simulink library "gbt_library"  (Simulink 7.4)
settings: Solver=ode45  StartTime=0.0  StopTime=10.0  RelTol=1e-3
undefined symbols (not defined in the file or in its folder): xlipgetpartsetting
libraries: xbsIndex_r4 x1348, casper_library_misc x29, casper_library_flow_control x4
(part 2 of 11)

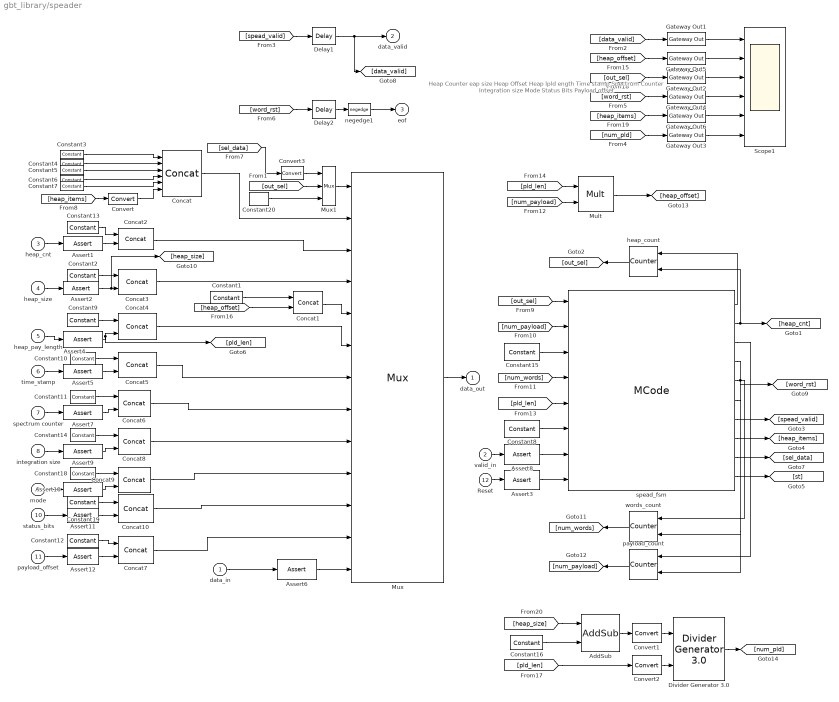
== system gbt_library/speader ==
  note: Heap Counter
      | eap size
      | Heap Offset
      | Heap lpld ength
      | Time stamp
      | Spectrum Counter
      | Integration size
      | Mode
      | Status Bits
      | Payload offset
  data_in : Inport
  valid_in : Inport  Port=2
  heap_cnt : Inport  Port=3
  heap_size : Inport  Port=4
  heap_pay_length : Inport  Port=5
  time_stamp : Inport  Port=6
  spectrum counter : Inport  Port=7
  integration size : Inport  Port=8
  mode : Inport  Port=9
  status_bits : Inport  Port=10
  payload_offset : Inport  Port=11
  Reset : Inport  Port=12
  AddSub : xbsIndex_r4/AddSub  mode=Subtraction  use_carryin=off  use_carryout=off  en=off  latency=0  precision=User Defined  arith_type=Unsigned  n_bits=40  bin_pt=0  quantization=Truncate  overflow=Wrap  dbl_ovrd=off  use_behavioral_HDL=off  hw_selection=Fabric  pipelined=off  block_type=addsub
  Assert{1..2,4..5,7,9..12} (9 alike) : xbsIndex_r4/Assert  assert_type=on  type_source=Explicitly  arith_type=Unsigned  n_bits=spead_lsw  bin_pt=0  assert_rate=off  rate_source=Explicitly  period=1  output_port=on  block_type=assert
      settings: block_version=11.4
  Assert3 : xbsIndex_r4/Assert  assert_type=on  type_source=Explicitly  arith_type=Boolean  n_bits=spead_lsw  bin_pt=0  assert_rate=on  rate_source=Explicitly  period=1  output_port=on  block_type=assert
      settings: block_version=11.4
  Assert6 : xbsIndex_r4/Assert  assert_type=on  type_source=Explicitly  arith_type=Unsigned  n_bits=64  bin_pt=0  assert_rate=off  rate_source=Explicitly  period=1  output_port=on  block_type=assert
      settings: block_version=11.4
  Assert8 : xbsIndex_r4/Assert  assert_type=on  type_source=Explicitly  arith_type=Boolean  n_bits=spead_lsw  bin_pt=0  assert_rate=on  rate_source=Explicitly  period=1  output_port=on  block_type=assert
      settings: block_version=11.4
  Concat : xbsIndex_r4/Concat  num_inputs=6  dbl_ovrd=off  block_type=concat
  Concat{1..10} (10 alike) : xbsIndex_r4/Concat  num_inputs=2  dbl_ovrd=off  block_type=concat
  Constant1 : xbsIndex_r4/Constant  arith_type=Unsigned  const=8388611  n_bits=spead_msw-spead_lsw  bin_pt=0  explicit_period=on  period=1  equ=P=C  opselect=C  inp2=PCIN>>17  opr=+  inp1=P  carry=CIN  dbl_ovrd=off  block_type=constant
      settings: block_version=11.4
  Constant10 : xbsIndex_r4/Constant  arith_type=Unsigned  const=8388628  n_bits=spead_msw-spead_lsw  bin_pt=0  explicit_period=on  period=1  equ=P=C  opselect=C  inp2=PCIN>>17  opr=+  inp1=P  carry=CIN  dbl_ovrd=off  block_type=constant
      settings: block_version=11.4
  Constant11 : xbsIndex_r4/Constant  arith_type=Unsigned  const=8388629  n_bits=spead_msw-spead_lsw  bin_pt=0  explicit_period=on  period=1  equ=P=C  opselect=C  inp2=PCIN>>17  opr=+  inp1=P  carry=CIN  dbl_ovrd=off  block_type=constant
      settings: block_version=11.4
  Constant12 : xbsIndex_r4/Constant  arith_type=Unsigned  const=26  n_bits=spead_msw-spead_lsw  bin_pt=0  explicit_period=on  period=1  equ=P=C  opselect=C  inp2=PCIN>>17  opr=+  inp1=P  carry=CIN  dbl_ovrd=off  block_type=constant
      settings: block_version=11.4
  Constant13 : xbsIndex_r4/Constant  arith_type=Unsigned  const=8388609  n_bits=spead_msw-spead_lsw  bin_pt=0  explicit_period=on  period=1  equ=P=C  opselect=C  inp2=PCIN>>17  opr=+  inp1=P  carry=CIN  dbl_ovrd=off  block_type=constant
      settings: block_version=11.4
  Constant14 : xbsIndex_r4/Constant  arith_type=Unsigned  const=8388630  n_bits=spead_msw-spead_lsw  bin_pt=0  explicit_period=on  period=1  equ=P=C  opselect=C  inp2=PCIN>>17  opr=+  inp1=P  carry=CIN  dbl_ovrd=off  block_type=constant
      settings: block_version=11.4
  Constant15 : xbsIndex_r4/Constant  arith_type=Unsigned  const=num_items+5  n_bits=8  bin_pt=0  explicit_period=on  period=1  equ=P=C  opselect=C  inp2=PCIN>>17  opr=+  inp1=P  carry=CIN  dbl_ovrd=off  block_type=constant
      settings: block_version=11.4
  Constant16 : xbsIndex_r4/Constant  arith_type=Unsigned  const=num_items*8  n_bits=8  bin_pt=0  explicit_period=on  period=1  equ=P=C  opselect=C  inp2=PCIN>>17  opr=+  inp1=P  carry=CIN  dbl_ovrd=off  block_type=constant
      settings: block_version=11.4
  Constant18 : xbsIndex_r4/Constant  arith_type=Unsigned  const=8388631  n_bits=spead_msw-spead_lsw  bin_pt=0  explicit_period=on  period=1  equ=P=C  opselect=C  inp2=PCIN>>17  opr=+  inp1=P  carry=CIN  dbl_ovrd=off  block_type=constant
      settings: block_version=11.4
  Constant19 : xbsIndex_r4/Constant  arith_type=Unsigned  const=8388632  n_bits=spead_msw-spead_lsw  bin_pt=0  explicit_period=on  period=1  equ=P=C  opselect=C  inp2=PCIN>>17  opr=+  inp1=P  carry=CIN  dbl_ovrd=off  block_type=constant
      settings: block_version=11.4
  Constant2 : xbsIndex_r4/Constant  arith_type=Unsigned  const=8388610  n_bits=spead_msw-spead_lsw  bin_pt=0  explicit_period=on  period=1  equ=P=C  opselect=C  inp2=PCIN>>17  opr=+  inp1=P  carry=CIN  dbl_ovrd=off  block_type=constant
      settings: block_version=11.4
  Constant20 : xbsIndex_r4/Constant  arith_type=Unsigned  const=num_items+5  n_bits=4  bin_pt=0  explicit_period=on  period=1  equ=P=C  opselect=C  inp2=PCIN>>17  opr=+  inp1=P  carry=CIN  dbl_ovrd=off  block_type=constant
      settings: block_version=11.4
  Constant3 : xbsIndex_r4/Constant  arith_type=Unsigned  const=83  n_bits=8  bin_pt=0  explicit_period=on  period=1  equ=P=C  opselect=C  inp2=PCIN>>17  opr=+  inp1=P  carry=CIN  dbl_ovrd=off  block_type=constant
      settings: block_version=11.4
  Constant4 : xbsIndex_r4/Constant  arith_type=Unsigned  const=4  n_bits=8  bin_pt=0  explicit_period=on  period=1  equ=P=C  opselect=C  inp2=PCIN>>17  opr=+  inp1=P  carry=CIN  dbl_ovrd=off  block_type=constant
      settings: block_version=11.4
  Constant5 : xbsIndex_r4/Constant  arith_type=Unsigned  const=3  n_bits=8  bin_pt=0  explicit_period=on  period=1  equ=P=C  opselect=C  inp2=PCIN>>17  opr=+  inp1=P  carry=CIN  dbl_ovrd=off  block_type=constant
      settings: block_version=11.4
  Constant6 : xbsIndex_r4/Constant  arith_type=Unsigned  const=5  n_bits=8  bin_pt=0  explicit_period=on  period=1  equ=P=C  opselect=C  inp2=PCIN>>17  opr=+  inp1=P  carry=CIN  dbl_ovrd=off  block_type=constant
      settings: block_version=11.4
  Constant7 : xbsIndex_r4/Constant  arith_type=Unsigned  const=0  n_bits=16  bin_pt=0  explicit_period=on  period=1  equ=P=C  opselect=C  inp2=PCIN>>17  opr=+  inp1=P  carry=CIN  dbl_ovrd=off  block_type=constant
      settings: block_version=11.4
  Constant8 : xbsIndex_r4/Constant  arith_type=Unsigned  const=2  n_bits=8  bin_pt=0  explicit_period=on  period=1  equ=P=C  opselect=C  inp2=PCIN>>17  opr=+  inp1=P  carry=CIN  dbl_ovrd=off  block_type=constant
      settings: block_version=11.4
  Constant9 : xbsIndex_r4/Constant  arith_type=Unsigned  const=8388612  n_bits=spead_msw-spead_lsw  bin_pt=0  explicit_period=on  period=1  equ=P=C  opselect=C  inp2=PCIN>>17  opr=+  inp1=P  carry=CIN  dbl_ovrd=off  block_type=constant
      settings: block_version=11.4
  Convert : xbsIndex_r4/Convert  arith_type=Unsigned  n_bits=16  bin_pt=0  quantization=Truncate  overflow=Wrap  latency=0  dbl_ovrd=off  pipeline=off  block_type=convert
      settings: block_version=11.4
  Convert1 : xbsIndex_r4/Convert  arith_type=Unsigned  n_bits=16  bin_pt=0  quantization=Truncate  overflow=Wrap  latency=0  dbl_ovrd=off  pipeline=off  block_type=convert
      settings: block_version=11.4
  Convert2 : xbsIndex_r4/Convert  arith_type=Unsigned  n_bits=16  bin_pt=0  quantization=Truncate  overflow=Wrap  latency=0  dbl_ovrd=off  pipeline=off  block_type=convert
      settings: block_version=11.4
  Convert3 : xbsIndex_r4/Convert  arith_type=Unsigned  n_bits=1  bin_pt=0  quantization=Truncate  overflow=Wrap  latency=0  dbl_ovrd=off  pipeline=off  block_type=convert
      settings: block_version=11.4
  Delay1 : xbsIndex_r4/Delay  en=off  latency=0  dbl_ovrd=off  reg_retiming=on  block_type=delay
      settings: block_version=11.4
  Delay2 : xbsIndex_r4/Delay  en=off  latency=0  dbl_ovrd=off  reg_retiming=on  block_type=delay
      settings: block_version=11.4
  "Divider Generator 3.0 " : xbsIndex_r4/Divider Generator 3.0   dividend_and_quotient_width=16  divisor_width=16  algorithm_type=Radix2  remainder_type=Remainder  fractional_width=16  clocks_per_division=1  divide_by_zero_detect=off  latency_configuration=Automatic  latency=20  ce=off  sclr=off  sclr_ce_priority=SCLR_overrides_CE  operand_sign=Signed  ip_name=Divider Generator  ip_version=3.0  dsptool_ready=true  wrapper_available=true  port_translation_map={ 'ce' => 'en', 'sclr' => 'rst' }  ipcore_fpga_part=xlipgetpartsetting(gcb, {'virtex4', 'xc4vsx35', '-10', 'ff668'})  ipcore_verbose=false  block_type=div_gen_v3_0
      settings: block_version=11.4
  Gateway Out{1..6} (6 alike) : xbsIndex_r4/Gateway Out  hdl_port=on  timing_constraint=None  locs_specified=off  LOCs={}  block_type=gatewayout
      settings: infoedit="Gateway out block.  Converts Xilinx fixed point inputs into ouputs of type Simulink integer, double, or fixed point.<br><br>Hardware notes:  In hardware these blocks become top level output ports or are discarded, depending on how they are configured."  block_version=11.4
  Mult : xbsIndex_r4/Mult  precision=User Defined  arith_type=Unsigned  n_bits=40  bin_pt=0  quantization=Truncate  overflow=Wrap  en=off  latency=1  dbl_ovrd=off  use_behavioral_HDL=off  opt=Speed  use_embedded=on  optimum_pipeline=off  pipeline=on  use_rpm=on  placement_style=Triangular  block_type=mult
      settings: block_version=11.4
  Mux : xbsIndex_r4/Mux  inputs=12  en=off  latency=0  precision=Full  arith_type="Signed  (2's comp)"  n_bits=8  bin_pt=2  quantization=Truncate  overflow=Wrap  dbl_ovrd=off  block_type=mux
      settings: block_version=11.4
  Mux1 : xbsIndex_r4/Mux  inputs=2  en=off  latency=0  precision=Full  arith_type="Signed  (2's comp)"  n_bits=8  bin_pt=2  quantization=Truncate  overflow=Wrap  dbl_ovrd=off  block_type=mux
      settings: block_version=11.4
  Scope1 : Scope  NumInputPorts=6
      settings: YMin=-5~-5~-5~-5~-5~-5  YMax=5~5~5~5~5~5  SaveName=ScopeData2  MaxDataPoints=10000
  heap_count : xbsIndex_r4/Counter  cnt_type=Free Running  cnt_to=Inf  operation=Up  start_count=0  cnt_by_val=1  arith_type=Unsigned  n_bits=4  bin_pt=0  load_pin=off  rst=on  en=on  explicit_period=on  period=1  dbl_ovrd=off  use_behavioral_HDL=off  implementation=Fabric  block_type=counter
      settings: block_version=11.4
  negedge1 : casper_library_misc/negedge  Tag=Rising Edge Detector  SystemSampleTime=-1
  payload_count : xbsIndex_r4/Counter  cnt_type=Free Running  cnt_to=Inf  operation=Up  start_count=0  cnt_by_val=1  arith_type=Unsigned  n_bits=8  bin_pt=0  load_pin=off  rst=on  en=on  explicit_period=on  period=1  dbl_ovrd=off  use_behavioral_HDL=off  implementation=Fabric  block_type=counter
      settings: block_version=11.4
  spead_fsm : xbsIndex_r4/MCode  mfname=spead_fsm  explicit_period=on  period=1  inputsTable={'boundInpExpr'=>['','','','5','','','','',''],'inputs'=>['head_count','num_payload_sent','total_header_len','min_header_len','num_words_sent','payload_len','total_num_payloads','data_valid_in','rst']}  outputsTable={'outputs'=>['head_count_rst','head_count_en','num_payload_rst','num_payload_en','words_sent_rst','words_sent_en','tge_valid','heap_elements','select_data','st'],'suppressOut'=>['off','off','off','off','off','off','off','off','off','off']}  dbl_ovrd=off  enable_stdout=off  enable_debug=off  suppress_output=on  defparams={'min_header_len',5}  hide_port_list={}  block_type=mcode
      settings: block_version=11.4
  words_count : xbsIndex_r4/Counter  cnt_type=Free Running  cnt_to=Inf  operation=Up  start_count=0  cnt_by_val=8  arith_type=Unsigned  n_bits=8  bin_pt=0  load_pin=off  rst=on  en=on  explicit_period=on  period=1  dbl_ovrd=off  use_behavioral_HDL=off  implementation=Fabric  block_type=counter
      settings: block_version=11.4
  data_out : Outport
  data_valid : Outport  Port=2
  eof : Outport  Port=3
  wires:
  Convert3/1 -> Mux1/1
  Convert2/1 -> "Divider Generator 3.0 "/2
  Convert1/1 -> "Divider Generator 3.0 "/1
  "Divider Generator 3.0 "/2 -> [num_pld]
  [pld_len] -> Convert2/1
  AddSub/1 -> Convert1/1
  Constant16/1 -> AddSub/2
  [heap_size] -> AddSub/1
  Delay2/1 -> negedge1/1
  Constant15/1 -> spead_fsm/3
  [num_words] -> spead_fsm/4
  [pld_len] -> spead_fsm/5
  Constant8/1 -> spead_fsm/6
  Assert8/1 -> spead_fsm/7
  Assert3/1 -> spead_fsm/8
  [word_rst] -> Delay2/1
  negedge1/1 -> eof/1
  Gateway Out5/1 -> Scope1/2
  [heap_offset] -> Gateway Out5/1
  Mult/1 -> [heap_offset]
  [pld_len] -> Mult/1
  [num_payload] -> Mult/2
  [num_payload] -> spead_fsm/2
  [out_sel] -> spead_fsm/1
  heap_count/1 -> [out_sel]
  payload_count/1 -> [num_payload]
  words_count/1 -> [num_words]
  Convert/1 -> Concat/6
  [heap_items] -> Convert/1
  [sel_data] -> Convert3/1
  spead_fsm/9 -> [sel_data]
  spead_fsm/10 -> [st]
  Mux1/1 -> Mux/1
  [out_sel] -> Mux1/2
  Constant20/1 -> Mux1/3
  [word_rst] -> Gateway Out4/1
  Gateway Out4/1 -> Scope1/4
  Gateway Out3/1 -> Scope1/6
  [num_pld] -> Gateway Out3/1
  Gateway Out1/1 -> Scope1/1
  [data_valid] -> Gateway Out1/1
  Reset/1 -> Assert3/1
  [heap_offset] -> Concat1/2
  valid_in/1 -> Assert8/1
  spead_fsm/8 -> [heap_items]
  spead_fsm/7 -> [spead_valid]
  spead_fsm/2 -> [heap_cnt], heap_count/2
  spead_fsm/1 -> heap_count/1
  spead_fsm/4 -> [word_rst], payload_count/2
  spead_fsm/3 -> payload_count/1
  spead_fsm/6 -> words_count/2
  spead_fsm/5 -> words_count/1
  Gateway Out6/1 -> Scope1/5
  Gateway Out2/1 -> Scope1/3
  Concat8/1 -> Mux/9
  Constant14/1 -> Concat8/1
  Assert9/1 -> Concat8/2
  integration size/1 -> Assert9/1
  Concat5/1 -> Mux/7
  Concat6/1 -> Mux/8
  Constant11/1 -> Concat6/1
  Assert7/1 -> Concat6/2
  spectrum counter/1 -> Assert7/1
  Concat9/1 -> Mux/10
  Concat10/1 -> Mux/11
  Concat7/1 -> Mux/12
  Assert6/1 -> Mux/13
  Concat1/1 -> Mux/5
  Constant1/1 -> Concat1/1
  [heap_items] -> Gateway Out6/1
  Delay1/1 -> [data_valid], data_valid/1
  [out_sel] -> Gateway Out2/1
  heap_pay_length/1 -> Assert4/1
  [spead_valid] -> Delay1/1
  Mux/1 -> data_out/1
  Concat2/1 -> Mux/3
  Assert5/1 -> Concat5/2
  Assert4/1 -> [pld_len], Concat4/2
  Assert2/1 -> [heap_size], Concat3/2
  Assert1/1 -> Concat2/2
  heap_cnt/1 -> Assert1/1
  heap_size/1 -> Assert2/1
  time_stamp/1 -> Assert5/1
  data_in/1 -> Assert6/1
  Constant10/1 -> Concat5/1
  Constant12/1 -> Concat7/1
  Constant13/1 -> Concat2/1
  Constant2/1 -> Concat3/1
  Constant3/1 -> Concat/1
  Constant4/1 -> Concat/2
  Constant5/1 -> Concat/3
  Constant6/1 -> Concat/4
  Constant7/1 -> Concat/5
  Constant9/1 -> Concat4/1
  Concat/1 -> Mux/2
  Concat3/1 -> Mux/4
  Concat4/1 -> Mux/6
  Constant18/1 -> Concat9/1
  mode/1 -> Assert10/1
  Assert10/1 -> Concat9/2
  Constant19/1 -> Concat10/1
  status_bits/1 -> Assert11/1
  Assert11/1 -> Concat10/2
  payload_offset/1 -> Assert12/1
  Assert12/1 -> Concat7/2

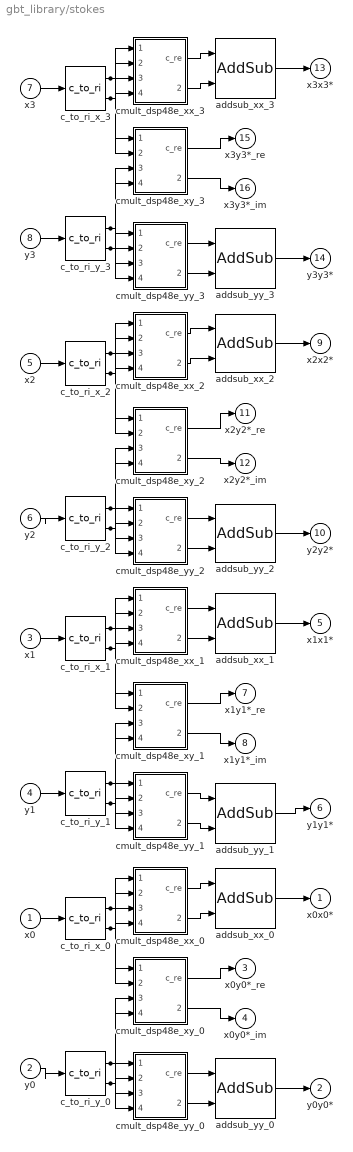
== system gbt_library/stokes ==
  x0 : Inport
  y0 : Inport  Port=2
  x1 : Inport  Port=3
  y1 : Inport  Port=4
  x2 : Inport  Port=5
  y2 : Inport  Port=6
  x3 : Inport  Port=7
  y3 : Inport  Port=8
  addsub_xx_{0..3} (4 alike) : xbsIndex_r4/AddSub  mode=Addition  use_carryin=off  use_carryout=off  en=off  latency=0  precision=Full  arith_type=Unsigned  n_bits=16  bin_pt=14  quantization=Truncate  overflow=Wrap  dbl_ovrd=off  use_behavioral_HDL=off  hw_selection=Fabric  pipelined=off  block_type=addsub
  addsub_yy_{0..3} (4 alike) : xbsIndex_r4/AddSub  mode=Addition  use_carryin=off  use_carryout=off  en=off  latency=0  precision=Full  arith_type=Unsigned  n_bits=16  bin_pt=14  quantization=Truncate  overflow=Wrap  dbl_ovrd=off  use_behavioral_HDL=off  hw_selection=Fabric  pipelined=off  block_type=addsub
  c_to_ri_x_{0..3} (4 alike) : casper_library_misc/c_to_ri  SystemSampleTime=-1  n_bits=18  bin_pt=0
      settings: AttributesFormatString=18_0 r/i
  c_to_ri_y_{0..3} (4 alike) : casper_library_misc/c_to_ri  SystemSampleTime=-1  n_bits=18  bin_pt=0
      settings: AttributesFormatString=18_0 r/i
  cmult_dsp48e_xx_0 : Subsystem  AncestorBlock=casper_library_multipliers/cmult_dsp48e  mask(cmult_dsp48e){n_bits_a=18, bin_pt_a=0, n_bits_b=18, bin_pt_b=0, conjugated=on, full_precision=on, n_bits_c=37, bin_pt_c=34, quantization=Truncate, overflow=Wrap, cast_latency=0}
      mask prompts: n_bits_a "Bit width 'a'"; bin_pt_a "Binary point 'a'"; n_bits_b "Bit width 'b'"; bin_pt_b "Binary point 'b'"; conjugated "Conjugate"; full_precision "Full precision"; n_bits_c "Bit width out"; bin_pt_c "Binary point out"; cast_latency "Cast Latency"
      mask help:
      | Multiplies two complex numbers using 4 DSP48Es.
      | Conjugation is optional.
      |
      | Re{a} and Im{a} can be up to 25 bits.
      | Re{b} and Im{b} can be up to 18 bits.
      mask init:
      | cmult_dsp48e_init(gcb, ...
      |     'n_bits_a', n_bits_a, ...
      |     'bin_pt_a', bin_pt_a, ...
      |     'n_bits_b', n_bits_b, ...
      |     'bin_pt_b', bin_pt_b, ...
      |     'conjugated', conjugated, ...
      |     'full_precision', full_precision, ...
      |     'n_bits_c', n_bits_c, ...
      |     'bin_pt_c', bin_pt_c, ...
      |     'quantization', quantization, ...
      |     'overflow', overflow, ...
      |     'cast_latency', cast_latency);
      settings: AttributesFormatString=|
      | 18_0 * 18_0 ==> 37_0
      | Latency=4
      mask StyleString: edit,edit,edit,edit,checkbox,checkbox,edit,edit,popup(Truncate|Round  (unbiased: +/- Inf)|Round  (unbiased: Even Values)),popup(Wrap|Saturate|Flag as error),edit
      mask CallbackString:
      | |||||full_precision = get_param(gcb, 'full_precision');
      | 
      | if strcmp(full_precision, 'on'),
      |     not_full_precision = 'off';
      | else
      |     not_full_precision = 'on';
      | end
      | 
      | set_param_state(gcb, 'n_bits_c', not_full_precision);
      | set_param_state(gcb, 'bin_pt_c', not_full_precision);
      | set_param_state(gcb, 'quantization', not_full_precision);
      | set_param_state(gcb, 'overflow', not_full_precision);
      | set_param_state(gcb, 'cast_latency', not_full_precision);|||||
      mask TabNameString: Basic,Basic,Basic,Basic,Basic,Output Type,Output Type,Output Type,Output Type,Output Type,Output Type
  cmult_dsp48e_xx_1 : Subsystem  AncestorBlock=casper_library_multipliers/cmult_dsp48e  mask(cmult_dsp48e){n_bits_a=18, bin_pt_a=0, n_bits_b=18, bin_pt_b=0, conjugated=on, full_precision=on, n_bits_c=37, bin_pt_c=34, quantization=Truncate, overflow=Wrap, cast_latency=0}
      mask prompts: n_bits_a "Bit width 'a'"; bin_pt_a "Binary point 'a'"; n_bits_b "Bit width 'b'"; bin_pt_b "Binary point 'b'"; conjugated "Conjugate"; full_precision "Full precision"; n_bits_c "Bit width out"; bin_pt_c "Binary point out"; cast_latency "Cast Latency"
      mask help:
      | Multiplies two complex numbers using 4 DSP48Es.
      | Conjugation is optional.
      |
      | Re{a} and Im{a} can be up to 25 bits.
      | Re{b} and Im{b} can be up to 18 bits.
      mask init: same as gbt_library/stokes/cmult_dsp48e_xx_0
      settings: AttributesFormatString=|
      | 18_0 * 18_0 ==> 37_0
      | Latency=4
      mask StyleString: edit,edit,edit,edit,checkbox,checkbox,edit,edit,popup(Truncate|Round  (unbiased: +/- Inf)|Round  (unbiased: Even Values)),popup(Wrap|Saturate|Flag as error),edit
      mask CallbackString:
      | |||||full_precision = get_param(gcb, 'full_precision');
      | 
      | if strcmp(full_precision, 'on'),
      |     not_full_precision = 'off';
      | else
      |     not_full_precision = 'on';
      | end
      | 
      | set_param_state(gcb, 'n_bits_c', not_full_precision);
      | set_param_state(gcb, 'bin_pt_c', not_full_precision);
      | set_param_state(gcb, 'quantization', not_full_precision);
      | set_param_state(gcb, 'overflow', not_full_precision);
      | set_param_state(gcb, 'cast_latency', not_full_precision);|||||
      mask TabNameString: Basic,Basic,Basic,Basic,Basic,Output Type,Output Type,Output Type,Output Type,Output Type,Output Type
  cmult_dsp48e_xx_2 : Subsystem  AncestorBlock=casper_library_multipliers/cmult_dsp48e  mask(cmult_dsp48e){n_bits_a=18, bin_pt_a=0, n_bits_b=18, bin_pt_b=0, conjugated=on, full_precision=on, n_bits_c=37, bin_pt_c=34, quantization=Truncate, overflow=Wrap, cast_latency=0}
      mask prompts: n_bits_a "Bit width 'a'"; bin_pt_a "Binary point 'a'"; n_bits_b "Bit width 'b'"; bin_pt_b "Binary point 'b'"; conjugated "Conjugate"; full_precision "Full precision"; n_bits_c "Bit width out"; bin_pt_c "Binary point out"; cast_latency "Cast Latency"
      mask help:
      | Multiplies two complex numbers using 4 DSP48Es.
      | Conjugation is optional.
      |
      | Re{a} and Im{a} can be up to 25 bits.
      | Re{b} and Im{b} can be up to 18 bits.
      mask init: same as gbt_library/stokes/cmult_dsp48e_xx_0
      settings: AttributesFormatString=|
      | 18_0 * 18_0 ==> 37_0
      | Latency=4
      mask StyleString: edit,edit,edit,edit,checkbox,checkbox,edit,edit,popup(Truncate|Round  (unbiased: +/- Inf)|Round  (unbiased: Even Values)),popup(Wrap|Saturate|Flag as error),edit
      mask CallbackString:
      | |||||full_precision = get_param(gcb, 'full_precision');
      | 
      | if strcmp(full_precision, 'on'),
      |     not_full_precision = 'off';
      | else
      |     not_full_precision = 'on';
      | end
      | 
      | set_param_state(gcb, 'n_bits_c', not_full_precision);
      | set_param_state(gcb, 'bin_pt_c', not_full_precision);
      | set_param_state(gcb, 'quantization', not_full_precision);
      | set_param_state(gcb, 'overflow', not_full_precision);
      | set_param_state(gcb, 'cast_latency', not_full_precision);|||||
      mask TabNameString: Basic,Basic,Basic,Basic,Basic,Output Type,Output Type,Output Type,Output Type,Output Type,Output Type
  cmult_dsp48e_xx_3 : Subsystem  AncestorBlock=casper_library_multipliers/cmult_dsp48e  mask(cmult_dsp48e){n_bits_a=18, bin_pt_a=0, n_bits_b=18, bin_pt_b=0, conjugated=on, full_precision=on, n_bits_c=37, bin_pt_c=34, quantization=Truncate, overflow=Wrap, cast_latency=0}
      mask prompts: n_bits_a "Bit width 'a'"; bin_pt_a "Binary point 'a'"; n_bits_b "Bit width 'b'"; bin_pt_b "Binary point 'b'"; conjugated "Conjugate"; full_precision "Full precision"; n_bits_c "Bit width out"; bin_pt_c "Binary point out"; cast_latency "Cast Latency"
      mask help:
      | Multiplies two complex numbers using 4 DSP48Es.
      | Conjugation is optional.
      |
      | Re{a} and Im{a} can be up to 25 bits.
      | Re{b} and Im{b} can be up to 18 bits.
      mask init: same as gbt_library/stokes/cmult_dsp48e_xx_0
      settings: AttributesFormatString=|
      | 18_0 * 18_0 ==> 37_0
      | Latency=4
      mask StyleString: edit,edit,edit,edit,checkbox,checkbox,edit,edit,popup(Truncate|Round  (unbiased: +/- Inf)|Round  (unbiased: Even Values)),popup(Wrap|Saturate|Flag as error),edit
      mask CallbackString:
      | |||||full_precision = get_param(gcb, 'full_precision');
      | 
      | if strcmp(full_precision, 'on'),
      |     not_full_precision = 'off';
      | else
      |     not_full_precision = 'on';
      | end
      | 
      | set_param_state(gcb, 'n_bits_c', not_full_precision);
      | set_param_state(gcb, 'bin_pt_c', not_full_precision);
      | set_param_state(gcb, 'quantization', not_full_precision);
      | set_param_state(gcb, 'overflow', not_full_precision);
      | set_param_state(gcb, 'cast_latency', not_full_precision);|||||
      mask TabNameString: Basic,Basic,Basic,Basic,Basic,Output Type,Output Type,Output Type,Output Type,Output Type,Output Type
  cmult_dsp48e_xy_0 : Subsystem  AncestorBlock=casper_library_multipliers/cmult_dsp48e  mask(cmult_dsp48e){n_bits_a=18, bin_pt_a=0, n_bits_b=18, bin_pt_b=0, conjugated=on, full_precision=on, n_bits_c=37, bin_pt_c=34, quantization=Truncate, overflow=Wrap, cast_latency=0}
      mask prompts: n_bits_a "Bit width 'a'"; bin_pt_a "Binary point 'a'"; n_bits_b "Bit width 'b'"; bin_pt_b "Binary point 'b'"; conjugated "Conjugate"; full_precision "Full precision"; n_bits_c "Bit width out"; bin_pt_c "Binary point out"; cast_latency "Cast Latency"
      mask help:
      | Multiplies two complex numbers using 4 DSP48Es.
      | Conjugation is optional.
      |
      | Re{a} and Im{a} can be up to 25 bits.
      | Re{b} and Im{b} can be up to 18 bits.
      mask init: same as gbt_library/stokes/cmult_dsp48e_xx_0
      settings: AttributesFormatString=|
      | 18_0 * 18_0 ==> 37_0
      | Latency=4
      mask StyleString: edit,edit,edit,edit,checkbox,checkbox,edit,edit,popup(Truncate|Round  (unbiased: +/- Inf)|Round  (unbiased: Even Values)),popup(Wrap|Saturate|Flag as error),edit
      mask CallbackString:
      | |||||full_precision = get_param(gcb, 'full_precision');
      | 
      | if strcmp(full_precision, 'on'),
      |     not_full_precision = 'off';
      | else
      |     not_full_precision = 'on';
      | end
      | 
      | set_param_state(gcb, 'n_bits_c', not_full_precision);
      | set_param_state(gcb, 'bin_pt_c', not_full_precision);
      | set_param_state(gcb, 'quantization', not_full_precision);
      | set_param_state(gcb, 'overflow', not_full_precision);
      | set_param_state(gcb, 'cast_latency', not_full_precision);|||||
      mask TabNameString: Basic,Basic,Basic,Basic,Basic,Output Type,Output Type,Output Type,Output Type,Output Type,Output Type
  cmult_dsp48e_xy_1 : Subsystem  AncestorBlock=casper_library_multipliers/cmult_dsp48e  mask(cmult_dsp48e){n_bits_a=18, bin_pt_a=0, n_bits_b=18, bin_pt_b=0, conjugated=on, full_precision=on, n_bits_c=37, bin_pt_c=34, quantization=Truncate, overflow=Wrap, cast_latency=0}
      mask prompts: n_bits_a "Bit width 'a'"; bin_pt_a "Binary point 'a'"; n_bits_b "Bit width 'b'"; bin_pt_b "Binary point 'b'"; conjugated "Conjugate"; full_precision "Full precision"; n_bits_c "Bit width out"; bin_pt_c "Binary point out"; cast_latency "Cast Latency"
      mask help:
      | Multiplies two complex numbers using 4 DSP48Es.
      | Conjugation is optional.
      |
      | Re{a} and Im{a} can be up to 25 bits.
      | Re{b} and Im{b} can be up to 18 bits.
      mask init: same as gbt_library/stokes/cmult_dsp48e_xx_0
      settings: AttributesFormatString=|
      | 18_0 * 18_0 ==> 37_0
      | Latency=4
      mask StyleString: edit,edit,edit,edit,checkbox,checkbox,edit,edit,popup(Truncate|Round  (unbiased: +/- Inf)|Round  (unbiased: Even Values)),popup(Wrap|Saturate|Flag as error),edit
      mask CallbackString:
      | |||||full_precision = get_param(gcb, 'full_precision');
      | 
      | if strcmp(full_precision, 'on'),
      |     not_full_precision = 'off';
      | else
      |     not_full_precision = 'on';
      | end
      | 
      | set_param_state(gcb, 'n_bits_c', not_full_precision);
      | set_param_state(gcb, 'bin_pt_c', not_full_precision);
      | set_param_state(gcb, 'quantization', not_full_precision);
      | set_param_state(gcb, 'overflow', not_full_precision);
      | set_param_state(gcb, 'cast_latency', not_full_precision);|||||
      mask TabNameString: Basic,Basic,Basic,Basic,Basic,Output Type,Output Type,Output Type,Output Type,Output Type,Output Type
  cmult_dsp48e_xy_2 : Subsystem  AncestorBlock=casper_library_multipliers/cmult_dsp48e  mask(cmult_dsp48e){n_bits_a=18, bin_pt_a=0, n_bits_b=18, bin_pt_b=0, conjugated=on, full_precision=on, n_bits_c=37, bin_pt_c=34, quantization=Truncate, overflow=Wrap, cast_latency=0}
      mask prompts: n_bits_a "Bit width 'a'"; bin_pt_a "Binary point 'a'"; n_bits_b "Bit width 'b'"; bin_pt_b "Binary point 'b'"; conjugated "Conjugate"; full_precision "Full precision"; n_bits_c "Bit width out"; bin_pt_c "Binary point out"; cast_latency "Cast Latency"
      mask help:
      | Multiplies two complex numbers using 4 DSP48Es.
      | Conjugation is optional.
      |
      | Re{a} and Im{a} can be up to 25 bits.
      | Re{b} and Im{b} can be up to 18 bits.
      mask init: same as gbt_library/stokes/cmult_dsp48e_xx_0
      settings: AttributesFormatString=|
      | 18_0 * 18_0 ==> 37_0
      | Latency=4
      mask StyleString: edit,edit,edit,edit,checkbox,checkbox,edit,edit,popup(Truncate|Round  (unbiased: +/- Inf)|Round  (unbiased: Even Values)),popup(Wrap|Saturate|Flag as error),edit
      mask CallbackString:
      | |||||full_precision = get_param(gcb, 'full_precision');
      | 
      | if strcmp(full_precision, 'on'),
      |     not_full_precision = 'off';
      | else
      |     not_full_precision = 'on';
      | end
      | 
      | set_param_state(gcb, 'n_bits_c', not_full_precision);
      | set_param_state(gcb, 'bin_pt_c', not_full_precision);
      | set_param_state(gcb, 'quantization', not_full_precision);
      | set_param_state(gcb, 'overflow', not_full_precision);
      | set_param_state(gcb, 'cast_latency', not_full_precision);|||||
      mask TabNameString: Basic,Basic,Basic,Basic,Basic,Output Type,Output Type,Output Type,Output Type,Output Type,Output Type
  cmult_dsp48e_xy_3 : Subsystem  AncestorBlock=casper_library_multipliers/cmult_dsp48e  mask(cmult_dsp48e){n_bits_a=18, bin_pt_a=0, n_bits_b=18, bin_pt_b=0, conjugated=on, full_precision=on, n_bits_c=37, bin_pt_c=34, quantization=Truncate, overflow=Wrap, cast_latency=0}
      mask prompts: n_bits_a "Bit width 'a'"; bin_pt_a "Binary point 'a'"; n_bits_b "Bit width 'b'"; bin_pt_b "Binary point 'b'"; conjugated "Conjugate"; full_precision "Full precision"; n_bits_c "Bit width out"; bin_pt_c "Binary point out"; cast_latency "Cast Latency"
      mask help:
      | Multiplies two complex numbers using 4 DSP48Es.
      | Conjugation is optional.
      |
      | Re{a} and Im{a} can be up to 25 bits.
      | Re{b} and Im{b} can be up to 18 bits.
      mask init: same as gbt_library/stokes/cmult_dsp48e_xx_0
      settings: AttributesFormatString=|
      | 18_0 * 18_0 ==> 37_0
      | Latency=4
      mask StyleString: edit,edit,edit,edit,checkbox,checkbox,edit,edit,popup(Truncate|Round  (unbiased: +/- Inf)|Round  (unbiased: Even Values)),popup(Wrap|Saturate|Flag as error),edit
      mask CallbackString:
      | |||||full_precision = get_param(gcb, 'full_precision');
      | 
      | if strcmp(full_precision, 'on'),
      |     not_full_precision = 'off';
      | else
      |     not_full_precision = 'on';
      | end
      | 
      | set_param_state(gcb, 'n_bits_c', not_full_precision);
      | set_param_state(gcb, 'bin_pt_c', not_full_precision);
      | set_param_state(gcb, 'quantization', not_full_precision);
      | set_param_state(gcb, 'overflow', not_full_precision);
      | set_param_state(gcb, 'cast_latency', not_full_precision);|||||
      mask TabNameString: Basic,Basic,Basic,Basic,Basic,Output Type,Output Type,Output Type,Output Type,Output Type,Output Type
  cmult_dsp48e_yy_0 : Subsystem  AncestorBlock=casper_library_multipliers/cmult_dsp48e  mask(cmult_dsp48e){n_bits_a=18, bin_pt_a=0, n_bits_b=18, bin_pt_b=0, conjugated=on, full_precision=on, n_bits_c=37, bin_pt_c=34, quantization=Truncate, overflow=Wrap, cast_latency=0}
      mask prompts: n_bits_a "Bit width 'a'"; bin_pt_a "Binary point 'a'"; n_bits_b "Bit width 'b'"; bin_pt_b "Binary point 'b'"; conjugated "Conjugate"; full_precision "Full precision"; n_bits_c "Bit width out"; bin_pt_c "Binary point out"; cast_latency "Cast Latency"
      mask help:
      | Multiplies two complex numbers using 4 DSP48Es.
      | Conjugation is optional.
      |
      | Re{a} and Im{a} can be up to 25 bits.
      | Re{b} and Im{b} can be up to 18 bits.
      mask init: same as gbt_library/stokes/cmult_dsp48e_xx_0
      settings: AttributesFormatString=|
      | 18_0 * 18_0 ==> 37_0
      | Latency=4
      mask StyleString: edit,edit,edit,edit,checkbox,checkbox,edit,edit,popup(Truncate|Round  (unbiased: +/- Inf)|Round  (unbiased: Even Values)),popup(Wrap|Saturate|Flag as error),edit
      mask CallbackString:
      | |||||full_precision = get_param(gcb, 'full_precision');
      | 
      | if strcmp(full_precision, 'on'),
      |     not_full_precision = 'off';
      | else
      |     not_full_precision = 'on';
      | end
      | 
      | set_param_state(gcb, 'n_bits_c', not_full_precision);
      | set_param_state(gcb, 'bin_pt_c', not_full_precision);
      | set_param_state(gcb, 'quantization', not_full_precision);
      | set_param_state(gcb, 'overflow', not_full_precision);
      | set_param_state(gcb, 'cast_latency', not_full_precision);|||||
      mask TabNameString: Basic,Basic,Basic,Basic,Basic,Output Type,Output Type,Output Type,Output Type,Output Type,Output Type
  cmult_dsp48e_yy_1 : Subsystem  AncestorBlock=casper_library_multipliers/cmult_dsp48e  mask(cmult_dsp48e){n_bits_a=18, bin_pt_a=0, n_bits_b=18, bin_pt_b=0, conjugated=on, full_precision=on, n_bits_c=37, bin_pt_c=34, quantization=Truncate, overflow=Wrap, cast_latency=0}
      mask prompts: n_bits_a "Bit width 'a'"; bin_pt_a "Binary point 'a'"; n_bits_b "Bit width 'b'"; bin_pt_b "Binary point 'b'"; conjugated "Conjugate"; full_precision "Full precision"; n_bits_c "Bit width out"; bin_pt_c "Binary point out"; cast_latency "Cast Latency"
      mask help:
      | Multiplies two complex numbers using 4 DSP48Es.
      | Conjugation is optional.
      |
      | Re{a} and Im{a} can be up to 25 bits.
      | Re{b} and Im{b} can be up to 18 bits.
      mask init: same as gbt_library/stokes/cmult_dsp48e_xx_0
      settings: AttributesFormatString=|
      | 18_0 * 18_0 ==> 37_0
      | Latency=4
      mask StyleString: edit,edit,edit,edit,checkbox,checkbox,edit,edit,popup(Truncate|Round  (unbiased: +/- Inf)|Round  (unbiased: Even Values)),popup(Wrap|Saturate|Flag as error),edit
      mask CallbackString:
      | |||||full_precision = get_param(gcb, 'full_precision');
      | 
      | if strcmp(full_precision, 'on'),
      |     not_full_precision = 'off';
      | else
      |     not_full_precision = 'on';
      | end
      | 
      | set_param_state(gcb, 'n_bits_c', not_full_precision);
      | set_param_state(gcb, 'bin_pt_c', not_full_precision);
      | set_param_state(gcb, 'quantization', not_full_precision);
      | set_param_state(gcb, 'overflow', not_full_precision);
      | set_param_state(gcb, 'cast_latency', not_full_precision);|||||
      mask TabNameString: Basic,Basic,Basic,Basic,Basic,Output Type,Output Type,Output Type,Output Type,Output Type,Output Type
  cmult_dsp48e_yy_2 : Subsystem  AncestorBlock=casper_library_multipliers/cmult_dsp48e  mask(cmult_dsp48e){n_bits_a=18, bin_pt_a=0, n_bits_b=18, bin_pt_b=0, conjugated=on, full_precision=on, n_bits_c=37, bin_pt_c=34, quantization=Truncate, overflow=Wrap, cast_latency=0}
      mask prompts: n_bits_a "Bit width 'a'"; bin_pt_a "Binary point 'a'"; n_bits_b "Bit width 'b'"; bin_pt_b "Binary point 'b'"; conjugated "Conjugate"; full_precision "Full precision"; n_bits_c "Bit width out"; bin_pt_c "Binary point out"; cast_latency "Cast Latency"
      mask help:
      | Multiplies two complex numbers using 4 DSP48Es.
      | Conjugation is optional.
      |
      | Re{a} and Im{a} can be up to 25 bits.
      | Re{b} and Im{b} can be up to 18 bits.
      mask init: same as gbt_library/stokes/cmult_dsp48e_xx_0
      settings: AttributesFormatString=|
      | 18_0 * 18_0 ==> 37_0
      | Latency=4
      mask StyleString: edit,edit,edit,edit,checkbox,checkbox,edit,edit,popup(Truncate|Round  (unbiased: +/- Inf)|Round  (unbiased: Even Values)),popup(Wrap|Saturate|Flag as error),edit
      mask CallbackString:
      | |||||full_precision = get_param(gcb, 'full_precision');
      | 
      | if strcmp(full_precision, 'on'),
      |     not_full_precision = 'off';
      | else
      |     not_full_precision = 'on';
      | end
      | 
      | set_param_state(gcb, 'n_bits_c', not_full_precision);
      | set_param_state(gcb, 'bin_pt_c', not_full_precision);
      | set_param_state(gcb, 'quantization', not_full_precision);
      | set_param_state(gcb, 'overflow', not_full_precision);
      | set_param_state(gcb, 'cast_latency', not_full_precision);|||||
      mask TabNameString: Basic,Basic,Basic,Basic,Basic,Output Type,Output Type,Output Type,Output Type,Output Type,Output Type
  cmult_dsp48e_yy_3 : Subsystem  AncestorBlock=casper_library_multipliers/cmult_dsp48e  mask(cmult_dsp48e){n_bits_a=18, bin_pt_a=0, n_bits_b=18, bin_pt_b=0, conjugated=on, full_precision=on, n_bits_c=37, bin_pt_c=34, quantization=Truncate, overflow=Wrap, cast_latency=0}
      mask prompts: n_bits_a "Bit width 'a'"; bin_pt_a "Binary point 'a'"; n_bits_b "Bit width 'b'"; bin_pt_b "Binary point 'b'"; conjugated "Conjugate"; full_precision "Full precision"; n_bits_c "Bit width out"; bin_pt_c "Binary point out"; cast_latency "Cast Latency"
      mask help:
      | Multiplies two complex numbers using 4 DSP48Es.
      | Conjugation is optional.
      |
      | Re{a} and Im{a} can be up to 25 bits.
      | Re{b} and Im{b} can be up to 18 bits.
      mask init: same as gbt_library/stokes/cmult_dsp48e_xx_0
      settings: AttributesFormatString=|
      | 18_0 * 18_0 ==> 37_0
      | Latency=4
      mask StyleString: edit,edit,edit,edit,checkbox,checkbox,edit,edit,popup(Truncate|Round  (unbiased: +/- Inf)|Round  (unbiased: Even Values)),popup(Wrap|Saturate|Flag as error),edit
      mask CallbackString:
      | |||||full_precision = get_param(gcb, 'full_precision');
      | 
      | if strcmp(full_precision, 'on'),
      |     not_full_precision = 'off';
      | else
      |     not_full_precision = 'on';
      | end
      | 
      | set_param_state(gcb, 'n_bits_c', not_full_precision);
      | set_param_state(gcb, 'bin_pt_c', not_full_precision);
      | set_param_state(gcb, 'quantization', not_full_precision);
      | set_param_state(gcb, 'overflow', not_full_precision);
      | set_param_state(gcb, 'cast_latency', not_full_precision);|||||
      mask TabNameString: Basic,Basic,Basic,Basic,Basic,Output Type,Output Type,Output Type,Output Type,Output Type,Output Type
  x0x0* : Outport
  y0y0* : Outport  Port=2
  x0y0*_re : Outport  Port=3
  x0y0*_im : Outport  Port=4
  x1x1* : Outport  Port=5
  y1y1* : Outport  Port=6
  x1y1*_re : Outport  Port=7
  x1y1*_im : Outport  Port=8
  x2x2* : Outport  Port=9
  y2y2* : Outport  Port=10
  x2y2*_re : Outport  Port=11
  x2y2*_im : Outport  Port=12
  x3x3* : Outport  Port=13
  y3y3* : Outport  Port=14
  x3y3*_re : Outport  Port=15
  x3y3*_im : Outport  Port=16
  wires:
  x0/1 -> c_to_ri_x_0/1
  y0/1 -> c_to_ri_y_0/1
  cmult_dsp48e_xy_0/1(c_re) -> x0y0*_re/1
  cmult_dsp48e_xy_0/2(c_im) -> x0y0*_im/1
  cmult_dsp48e_xx_0/1(c_re) -> addsub_xx_0/1
  cmult_dsp48e_xx_0/2(c_im) -> addsub_xx_0/2
  addsub_xx_0/1 -> x0x0*/1
  cmult_dsp48e_yy_0/1(c_re) -> addsub_yy_0/1
  cmult_dsp48e_yy_0/2(c_im) -> addsub_yy_0/2
  addsub_yy_0/1 -> y0y0*/1
  x1/1 -> c_to_ri_x_1/1
  y1/1 -> c_to_ri_y_1/1
  cmult_dsp48e_xy_1/1(c_re) -> x1y1*_re/1
  cmult_dsp48e_xy_1/2(c_im) -> x1y1*_im/1
  cmult_dsp48e_xx_1/1(c_re) -> addsub_xx_1/1
  cmult_dsp48e_xx_1/2(c_im) -> addsub_xx_1/2
  addsub_xx_1/1 -> x1x1*/1
  cmult_dsp48e_yy_1/1(c_re) -> addsub_yy_1/1
  cmult_dsp48e_yy_1/2(c_im) -> addsub_yy_1/2
  addsub_yy_1/1 -> y1y1*/1
  x2/1 -> c_to_ri_x_2/1
  y2/1 -> c_to_ri_y_2/1
  cmult_dsp48e_xy_2/1(c_re) -> x2y2*_re/1
  cmult_dsp48e_xy_2/2(c_im) -> x2y2*_im/1
  cmult_dsp48e_xx_2/1(c_re) -> addsub_xx_2/1
  cmult_dsp48e_xx_2/2(c_im) -> addsub_xx_2/2
  addsub_xx_2/1 -> x2x2*/1
  cmult_dsp48e_yy_2/1(c_re) -> addsub_yy_2/1
  cmult_dsp48e_yy_2/2(c_im) -> addsub_yy_2/2
  addsub_yy_2/1 -> y2y2*/1
  x3/1 -> c_to_ri_x_3/1
  y3/1 -> c_to_ri_y_3/1
  cmult_dsp48e_xy_3/1(c_re) -> x3y3*_re/1
  cmult_dsp48e_xy_3/2(c_im) -> x3y3*_im/1
  cmult_dsp48e_xx_3/1(c_re) -> addsub_xx_3/1
  cmult_dsp48e_xx_3/2(c_im) -> addsub_xx_3/2
  addsub_xx_3/1 -> x3x3*/1
  cmult_dsp48e_yy_3/1(c_re) -> addsub_yy_3/1
  cmult_dsp48e_yy_3/2(c_im) -> addsub_yy_3/2
  addsub_yy_3/1 -> y3y3*/1
  c_to_ri_y_3/2 -> cmult_dsp48e_yy_3/2(a_im), cmult_dsp48e_yy_3/4(b_im), cmult_dsp48e_xy_3/4(b_im)
  c_to_ri_y_3/1 -> cmult_dsp48e_yy_3/1(a_re), cmult_dsp48e_yy_3/3(b_re), cmult_dsp48e_xy_3/3(b_re)
  c_to_ri_x_3/2 -> cmult_dsp48e_xx_3/2(a_im), cmult_dsp48e_xx_3/4(b_im), cmult_dsp48e_xy_3/2(a_im)
  c_to_ri_x_3/1 -> cmult_dsp48e_xx_3/1(a_re), cmult_dsp48e_xx_3/3(b_re), cmult_dsp48e_xy_3/1(a_re)
  c_to_ri_y_2/2 -> cmult_dsp48e_yy_2/2(a_im), cmult_dsp48e_yy_2/4(b_im), cmult_dsp48e_xy_2/4(b_im)
  c_to_ri_y_2/1 -> cmult_dsp48e_yy_2/1(a_re), cmult_dsp48e_yy_2/3(b_re), cmult_dsp48e_xy_2/3(b_re)
  c_to_ri_x_2/2 -> cmult_dsp48e_xx_2/2(a_im), cmult_dsp48e_xx_2/4(b_im), cmult_dsp48e_xy_2/2(a_im)
  c_to_ri_x_2/1 -> cmult_dsp48e_xx_2/1(a_re), cmult_dsp48e_xx_2/3(b_re), cmult_dsp48e_xy_2/1(a_re)
  c_to_ri_y_1/2 -> cmult_dsp48e_yy_1/2(a_im), cmult_dsp48e_yy_1/4(b_im), cmult_dsp48e_xy_1/4(b_im)
  c_to_ri_y_1/1 -> cmult_dsp48e_yy_1/1(a_re), cmult_dsp48e_yy_1/3(b_re), cmult_dsp48e_xy_1/3(b_re)
  c_to_ri_x_1/2 -> cmult_dsp48e_xx_1/2(a_im), cmult_dsp48e_xx_1/4(b_im), cmult_dsp48e_xy_1/2(a_im)
  c_to_ri_x_1/1 -> cmult_dsp48e_xx_1/1(a_re), cmult_dsp48e_xx_1/3(b_re), cmult_dsp48e_xy_1/1(a_re)
  c_to_ri_y_0/2 -> cmult_dsp48e_yy_0/2(a_im), cmult_dsp48e_yy_0/4(b_im), cmult_dsp48e_xy_0/4(b_im)
  c_to_ri_y_0/1 -> cmult_dsp48e_yy_0/1(a_re), cmult_dsp48e_yy_0/3(b_re), cmult_dsp48e_xy_0/3(b_re)
  c_to_ri_x_0/2 -> cmult_dsp48e_xx_0/2(a_im), cmult_dsp48e_xx_0/4(b_im), cmult_dsp48e_xy_0/2(a_im)
  c_to_ri_x_0/1 -> cmult_dsp48e_xx_0/1(a_re), cmult_dsp48e_xx_0/3(b_re), cmult_dsp48e_xy_0/1(a_re)

== system gbt_library/Parallel_CIC_filter/Stage1_dec5 ==
  sync_in : Inport
  in1 : Inport  Port=2
  in2 : Inport  Port=3
  in3 : Inport  Port=4
  in4 : Inport  Port=5
  decimator_5 : Subsystem
  p_adder1 : Subsystem
  p_adder2 : Subsystem
  p_adder3 : Subsystem
  sync_out : Outport
  out1 : Outport  Port=2
  out2 : Outport  Port=3
  out3 : Outport  Port=4
  out4 : Outport  Port=5
  wires:
  decimator_5/5(Out4) -> out4/1
  decimator_5/4(Out3) -> out3/1
  decimator_5/3(Out2) -> out2/1
  decimator_5/2(Out1) -> out1/1
  decimator_5/1(sync_out) -> sync_out/1
  p_adder3/5(out4) -> decimator_5/5(In4)  "pa_i4_4"
  p_adder3/4(out3) -> decimator_5/4(In3)  "pa_i4_3"
  p_adder3/3(out2) -> decimator_5/3(In2)  "pa_i4_2"
  p_adder3/2(out1) -> decimator_5/2(In1)  "pa_i4_1"
  p_adder3/1(sync_out) -> decimator_5/1(sync_in)  "sync_in4"
  p_adder2/5(out4) -> p_adder3/5(in4)  "pa_i3_4"
  p_adder2/4(out3) -> p_adder3/4(in3)  "pa_i3_3"
  p_adder2/3(out2) -> p_adder3/3(in2)  "pa_i3_2"
  p_adder2/2(out1) -> p_adder3/2(in1)  "pa_i3_1"
  p_adder2/1(sync_out) -> p_adder3/1(sync_in)  "sync_in3"
  p_adder1/5(out4) -> p_adder2/5(in4)  "pa_i2_4"
  p_adder1/4(out3) -> p_adder2/4(in3)  "pa_i2_3"
  p_adder1/3(out2) -> p_adder2/3(in2)  "pa_i2_2"
  p_adder1/2(out1) -> p_adder2/2(in1)  "pa_i2_1"
  p_adder1/1(sync_out) -> p_adder2/1(sync_in)  "sync_in2"
  in4/1 -> p_adder1/5(in4)
  in3/1 -> p_adder1/4(in3)
  in2/1 -> p_adder1/3(in2)
  in1/1 -> p_adder1/2(in1)
  sync_in/1 -> p_adder1/1(sync_in)

== system gbt_library/Parallel_CIC_filter/Stage2_dec5 ==
  sync_in : Inport
  in1 : Inport  Port=2
  in2 : Inport  Port=3
  in3 : Inport  Port=4
  in4 : Inport  Port=5
  decimator_5 : Subsystem
  p_adder1 : Subsystem
  p_adder2 : Subsystem
  p_adder3 : Subsystem
  sync_out : Outport
  out1 : Outport  Port=2
  out2 : Outport  Port=3
  out3 : Outport  Port=4
  out4 : Outport  Port=5
  wires:
  decimator_5/5(Out4) -> out4/1
  decimator_5/4(Out3) -> out3/1
  decimator_5/3(Out2) -> out2/1
  decimator_5/2(Out1) -> out1/1
  decimator_5/1(sync_out) -> sync_out/1
  p_adder3/5(out4) -> decimator_5/5(In4)  "pa_i4_4"
  p_adder3/4(out3) -> decimator_5/4(In3)  "pa_i4_3"
  p_adder3/3(out2) -> decimator_5/3(In2)  "pa_i4_2"
  p_adder3/2(out1) -> decimator_5/2(In1)  "pa_i4_1"
  p_adder3/1(sync_out) -> decimator_5/1(sync_in)  "sync_in4"
  p_adder2/5(out4) -> p_adder3/5(in4)  "pa_i3_4"
  p_adder2/4(out3) -> p_adder3/4(in3)  "pa_i3_3"
  p_adder2/3(out2) -> p_adder3/3(in2)  "pa_i3_2"
  p_adder2/2(out1) -> p_adder3/2(in1)  "pa_i3_1"
  p_adder2/1(sync_out) -> p_adder3/1(sync_in)  "sync_in3"
  p_adder1/5(out4) -> p_adder2/5(in4)  "pa_i2_4"
  p_adder1/4(out3) -> p_adder2/4(in3)  "pa_i2_3"
  p_adder1/3(out2) -> p_adder2/3(in2)  "pa_i2_2"
  p_adder1/2(out1) -> p_adder2/2(in1)  "pa_i2_1"
  p_adder1/1(sync_out) -> p_adder2/1(sync_in)  "sync_in2"
  in4/1 -> p_adder1/5(in4)
  in3/1 -> p_adder1/4(in3)
  in2/1 -> p_adder1/3(in2)
  in1/1 -> p_adder1/2(in1)
  sync_in/1 -> p_adder1/1(sync_in)

== system gbt_library/Parallel_CIC_filter/Stage3_dec2 ==
  sync_in : Inport
  in1 : Inport  Port=2
  in2 : Inport  Port=3
  in3 : Inport  Port=4
  in4 : Inport  Port=5
  p_adder1 : Subsystem
  p_adder2 : Subsystem
  p_adder3 : Subsystem
  sync_out : Outport
  out1 : Outport  Port=2
  out2 : Outport  Port=3
  wires:
  p_adder3/5(out4) -> out2/1  "pa_i4_4"
  p_adder3/3(out2) -> out1/1  "pa_i4_2"
  p_adder3/1(sync_out) -> sync_out/1  "sync_in4"
  p_adder2/5(out4) -> p_adder3/5(in4)  "pa_i3_4"
  p_adder2/4(out3) -> p_adder3/4(in3)  "pa_i3_3"
  p_adder2/3(out2) -> p_adder3/3(in2)  "pa_i3_2"
  p_adder2/2(out1) -> p_adder3/2(in1)  "pa_i3_1"
  p_adder2/1(sync_out) -> p_adder3/1(sync_in)  "sync_in3"
  p_adder1/5(out4) -> p_adder2/5(in4)  "pa_i2_4"
  p_adder1/4(out3) -> p_adder2/4(in3)  "pa_i2_3"
  p_adder1/3(out2) -> p_adder2/3(in2)  "pa_i2_2"
  p_adder1/2(out1) -> p_adder2/2(in1)  "pa_i2_1"
  p_adder1/1(sync_out) -> p_adder2/1(sync_in)  "sync_in2"
  in4/1 -> p_adder1/5(in4)
  in3/1 -> p_adder1/4(in3)
  in2/1 -> p_adder1/3(in2)
  in1/1 -> p_adder1/2(in1)
  sync_in/1 -> p_adder1/1(sync_in)

== system gbt_library/Parallel_CIC_filter/Stage4_dec2 ==
  sync_in : Inport
  in1 : Inport  Port=2
  in2 : Inport  Port=3
  p_adder1 : Subsystem
  p_adder2 : Subsystem
  p_adder3 : Subsystem
  sync_out : Outport
  out1 : Outport  Port=2
  wires:
  p_adder3/3(out2) -> out1/1  "pa_i4_2"
  p_adder3/1(sync_out) -> sync_out/1  "sync_in4"
  p_adder2/3(out2) -> p_adder3/3(in2)  "pa_i3_2"
  p_adder2/2(out1) -> p_adder3/2(in1)  "pa_i3_1"
  p_adder2/1(sync_out) -> p_adder3/1(sync_in)  "sync_in3"
  p_adder1/3(out2) -> p_adder2/3(in2)  "pa_i2_2"
  p_adder1/2(out1) -> p_adder2/2(in1)  "pa_i2_1"
  p_adder1/1(sync_out) -> p_adder2/1(sync_in)  "sync_in2"
  in2/1 -> p_adder1/3(in2)
  in1/1 -> p_adder1/2(in1)
  sync_in/1 -> p_adder1/1(sync_in)

== system gbt_library/Parallel_CIC_filter_stage/decimator_7 ==
  sync_in : Inport
  In1 : Inport  Port=2
  In2 : Inport  Port=3
  In3 : Inport  Port=4
  In4 : Inport  Port=5
  Down_sample{1..4} (4 alike) : xbsIndex_r4/Down Sample  sample_ratio=7  sample_phase="Last Value of Frame  (most efficient)"  en=off  latency=1  dbl_ovrd=off  block_type=dsamp
      settings: block_version=11.4
  delay1 : xbsIndex_r4/Delay  en=off  latency=5  dbl_ovrd=off  reg_retiming=off  block_type=delay
      settings: block_version=11.4
  delay2 : xbsIndex_r4/Delay  en=off  latency=0  dbl_ovrd=off  reg_retiming=off  block_type=delay
      settings: block_version=11.4
  delay3 : xbsIndex_r4/Delay  en=off  latency=2  dbl_ovrd=off  reg_retiming=off  block_type=delay
      settings: block_version=11.4
  delay4 : xbsIndex_r4/Delay  en=off  latency=4  dbl_ovrd=off  reg_retiming=off  block_type=delay
      settings: block_version=11.4
  sync_delay : xbsIndex_r4/Delay  en=off  latency=1  dbl_ovrd=off  reg_retiming=off  block_type=delay
      settings: block_version=11.4
  sync_out : Outport
  Out1 : Outport  Port=2
  Out2 : Outport  Port=3
  Out3 : Outport  Port=4
  Out4 : Outport  Port=5
  wires:
  sync_delay/1 -> sync_out/1
  sync_in/1 -> sync_delay/1
  Down_sample4/1 -> Out2/1
  delay4/1 -> Down_sample4/1  "dO4"
  In4/1 -> delay4/1
  Down_sample3/1 -> Out3/1
  delay3/1 -> Down_sample3/1  "dO3"
  In3/1 -> delay3/1
  Down_sample2/1 -> Out4/1
  delay2/1 -> Down_sample2/1  "dO2"
  In2/1 -> delay2/1
  Down_sample1/1 -> Out1/1
  delay1/1 -> Down_sample1/1  "dO1"
  In1/1 -> delay1/1

== system gbt_library/Parallel_CIC_filter_stage/p_adder1 ==
  sync_in : Inport
  in1 : Inport  Port=2
  in2 : Inport  Port=3
  in3 : Inport  Port=4
  in4 : Inport  Port=5
  adder_tree1 : Subsystem
  adder_tree2 : Subsystem
  adder_tree3 : Subsystem
  adder_tree4 : Subsystem
  delay1_{1..4} (4 alike) : xbsIndex_r4/Delay  en=off  latency=1  dbl_ovrd=off  reg_retiming=off  block_type=delay
      settings: block_version=11.4
  sync_out : Outport
  out1 : Outport  Port=2
  out2 : Outport  Port=3
  out3 : Outport  Port=4
  out4 : Outport  Port=5
  wires:
  in1/1 -> adder_tree4/5(din_4), adder_tree3/4(din_3), adder_tree2/3(din_2), adder_tree1/2(din_1), delay1_1/1
  in2/1 -> adder_tree4/4(din_3), adder_tree3/3(din_2), adder_tree2/2(din_1), delay1_2/1
  in3/1 -> adder_tree4/3(din_2), adder_tree3/2(din_1), delay1_3/1
  in4/1 -> adder_tree4/2(din_1), delay1_4/1
  delay1_4/1 -> adder_tree4/6(din_5), adder_tree3/5(din_4), adder_tree2/4(din_3), adder_tree1/3(din_2)  "d1_4"
  delay1_3/1 -> adder_tree4/7(din_6), adder_tree3/6(din_5), adder_tree2/5(din_4), adder_tree1/4(din_3)  "d1_3"
  delay1_2/1 -> adder_tree4/8(din_7), adder_tree3/7(din_6), adder_tree2/6(din_5), adder_tree1/5(din_4)  "d1_2"
  delay1_1/1 -> adder_tree3/8(din_7), adder_tree2/7(din_6), adder_tree1/6(din_5)  "d1_1"
  adder_tree4/1(sync_out) -> sync_out/1  "adder_tree_sync_in4"
  adder_tree4/2(dout) -> out4/1
  adder_tree3/1(sync_out) -> adder_tree4/1(sync)  "adder_tree_sync_in3"
  adder_tree3/2(dout) -> out3/1
  adder_tree2/1(sync_out) -> adder_tree3/1(sync)  "adder_tree_sync_in2"
  adder_tree2/2(dout) -> out2/1
  adder_tree1/1(sync_out) -> adder_tree2/1(sync)  "adder_tree_sync_in1"
  adder_tree1/2(dout) -> out1/1
  sync_in/1 -> adder_tree1/1(sync)
